simulink model "Quat"  (R2022b)
settings: Solver=FixedStepAuto  StartTime=0.0  StopTime=10.0  RelTol=1e-3
settings Model: Creator=yuzehong  LastModifiedBy=程一帆
settings OptimizationCC: DefaultParameterBehavior=Inlined  UseDivisionForNetSlopeComputation=on  GainParamInheritBuiltInType=on  UseFloatMulNetSlope=on  InlineInvariantSignals=on  ReuseModelBlockBuffer=on  PassReuseOutputArgsAs=Individual arguments  NoFixptDivByZeroProtection=on  EfficientFloat2IntCast=on  LifeSpan=1  OptimizeBlockOrder=speed  DifferentSizesBufferReuse=on  EfficientTunableParamExpr=on
settings DebuggingCC: ParameterTunabilityLossMsg=error
settings HardwareCC: ProdLongLongMode=on
settings SFSimCC: MATLABDynamicMemAlloc=off
settings RTWCC: Description=Embedded Coder  SystemTargetFile=ert.tlc  GenCodeOnly=on  TemplateMakefile=ert_default_tmf  GPUComputeCapability=5.0
settings CodeAppCC: GenerateComments=off  IgnoreCustomStorageClasses=off  OperatorAnnotations=on  SimulinkDataObjDesc=on  SFDataObjDesc=on  CustomSymbolStrGlobalVar=rt$N$M  CustomSymbolStrType=$N$M  CustomSymbolStrFcn=$N$M$F  CustomSymbolStrMacro=$N$M  SimulinkBlockComments=off
settings ERTTargetCC: TargetLangStandard=C99 (ISO)  GenerateSampleERTMain=on  IncludeMdlTerminateFcn=off  CombineSignalStateStructs=on  SupportAbsoluteTime=off  CodeInterfacePackaging=Reusable function  SupportComplex=off  SupportContinuousTime=on  InlinedParameterPlacement=NonHierarchical  ERTCustomFileTemplate=example_file_process.tlc  ERTFilePackagingFormat=CompactWithDataFile

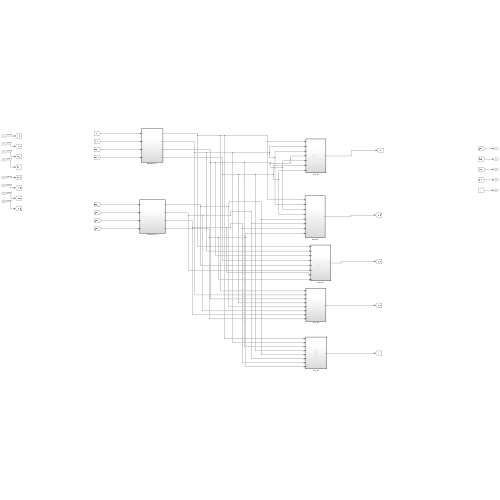
[thumbnail: Simulink's stored preview of the top-level diagram]
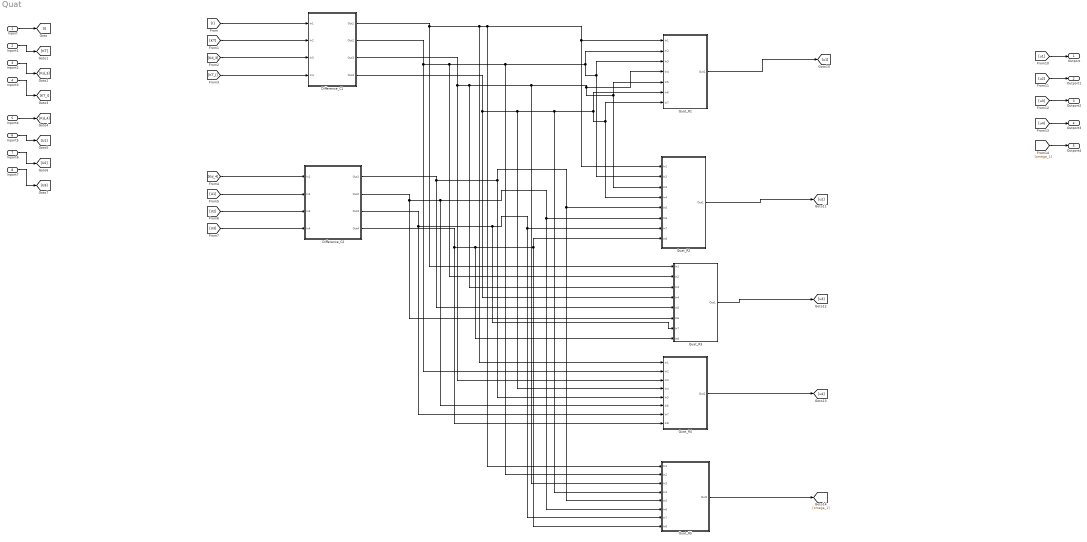
== system Quat ==
  Inport : Inport  OutDataTypeStr=int32  PortDimensions=8
  Inport1 : Inport  Port=2  OutDataTypeStr=int32  PortDimensions=8
  Inport2 : Inport  Port=3  OutDataTypeStr=int32  PortDimensions=8
  Inport3 : Inport  Port=4  OutDataTypeStr=int32  PortDimensions=8
  Inport4 : Inport  Port=5  OutDataTypeStr=int32  PortDimensions=8
  Inport5 : Inport  Port=6  OutDataTypeStr=int32  PortDimensions=8
  Inport6 : Inport  Port=7  OutDataTypeStr=int32  PortDimensions=8
  Inport7 : Inport  Port=8  OutDataTypeStr=int32  PortDimensions=8
  Difference_C1 : Subsystem  TreatAsAtomicUnit=on
      settings: RTWFcnNameOpts=Use subsystem name
  Difference_C2 : Subsystem  TreatAsAtomicUnit=on
      settings: RTWFcnNameOpts=Use subsystem name
  Quat_R1 : Subsystem  TreatAsAtomicUnit=on
      settings: RTWFcnNameOpts=Use subsystem name
  Quat_R2 : Subsystem  TreatAsAtomicUnit=on
      settings: RTWFcnNameOpts=Use subsystem name
  Quat_R3 : Subsystem  TreatAsAtomicUnit=on
      settings: RTWFcnNameOpts=Use subsystem name
  Quat_R4 : Subsystem  TreatAsAtomicUnit=on
      settings: RTWFcnNameOpts=Use subsystem name
  Quat_R5 : Subsystem  TreatAsAtomicUnit=on
      settings: RTWFcnNameOpts=Use subsystem name
  Outport : Outport
  Outport1 : Outport  Port=2
  Outport2 : Outport  Port=3
  Outport3 : Outport  Port=4
  Outport4 : Outport  Port=5
  wires:
  Quat_R1/1(Out1) -> [u1]
  Quat_R2/1(Out1) -> [u2]
  Quat_R3/1(Out1) -> [u3]
  Quat_R4/1(Out1) -> [u4]
  Quat_R5/1(Out1) -> [omega_1]
  Difference_C1/3(Out3) -> Quat_R4/3(In3), Quat_R3/3(In3), Quat_R5/3(In3), Quat_R1/4(In4), Quat_R2/3(In3), Quat_R1/5(In5)
  Difference_C1/2(Out2) -> Quat_R4/2(In2), Quat_R3/2(In2), Quat_R5/2(In2), Quat_R1/2(In2), Quat_R2/2(In2), Quat_R1/3(In3)
  Difference_C1/4(Out4) -> Quat_R3/4(In4), Quat_R4/4(In4), Quat_R5/4(In4), Quat_R1/6(In6), Quat_R2/4(In4), Quat_R1/7(In7)
  Difference_C1/1(Out1) -> Quat_R3/1(In1), Quat_R4/1(In1), Quat_R5/1(In1), Quat_R2/1(In1), Quat_R1/1(In1)
  [I] -> Difference_C1/1(In1)
  [KT] -> Difference_C1/2(In2)
  [Kd_3] -> Difference_C1/3(In3)
  [KT_I] -> Difference_C1/4(In4)
  Difference_C2/4(Out4) -> Quat_R4/8(In8), Quat_R3/8(In8), Quat_R5/8(In8), Quat_R2/8(In8)
  Difference_C2/2(Out2) -> Quat_R3/6(In6), Quat_R4/6(In6), Quat_R5/6(In6), Quat_R2/6(In6)
  Difference_C2/3(Out3) -> Quat_R4/7(In7), Quat_R3/7(In7), Quat_R5/7(In7), Quat_R2/7(In7)
  Difference_C2/1(Out1) -> Quat_R3/5(In5), Quat_R4/5(In5), Quat_R5/5(In5), Quat_R2/5(In5)
  [Kd_4] -> Difference_C2/1(In1)
  [U1] -> Difference_C2/2(In2)
  [U2] -> Difference_C2/3(In3)
  [U3] -> Difference_C2/4(In4)
  Inport/1 -> [I]
  Inport1/1 -> [KT]
  Inport2/1 -> [Kd_3]
  Inport3/1 -> [KT_I]
  Inport4/1 -> [Kd_4]
  Inport5/1 -> [U1]
  Inport6/1 -> [U2]
  Inport7/1 -> [U3]
  [u1] -> Outport/1
  [u2] -> Outport1/1
  [u3] -> Outport2/1
  [u4] -> Outport3/1
  [omega_1] -> Outport4/1

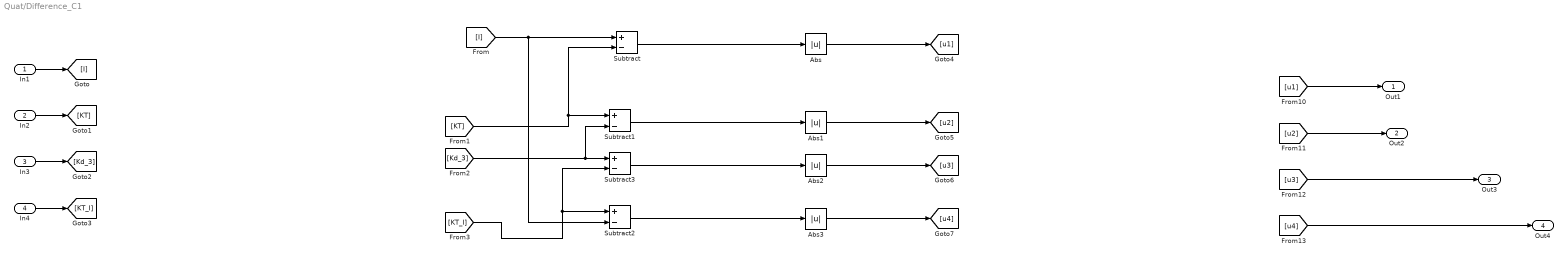
== system Quat/Difference_C1 ==
  In1 : Inport
  In2 : Inport  Port=2
  In3 : Inport  Port=3
  In4 : Inport  Port=4
  Abs{,1..3} (4 alike) : Abs  SaturateOnIntegerOverflow=off
  Subtract{,1..3} (4 alike) : Sum  Inputs=+-
  Out1 : Outport
  Out2 : Outport  Port=2
  Out3 : Outport  Port=3
  Out4 : Outport  Port=4
  wires:
  [KT_I] -> Subtract3/2, Subtract2/1
  Subtract2/1 -> Abs3/1
  [I] -> Subtract2/2, Subtract/1
  [Kd_3] -> Subtract1/2, Subtract3/1
  Subtract1/1 -> Abs1/1
  [KT] -> Subtract/2, Subtract1/1
  Subtract/1 -> Abs/1
  Abs1/1 -> [u2]
  Subtract3/1 -> Abs2/1
  Abs/1 -> [u1]
  In1/1 -> [I]
  In2/1 -> [KT]
  In3/1 -> [Kd_3]
  In4/1 -> [KT_I]
  [u3] -> Out3/1
  [u4] -> Out4/1
  [u1] -> Out1/1
  [u2] -> Out2/1
  Abs2/1 -> [u3]
  Abs3/1 -> [u4]

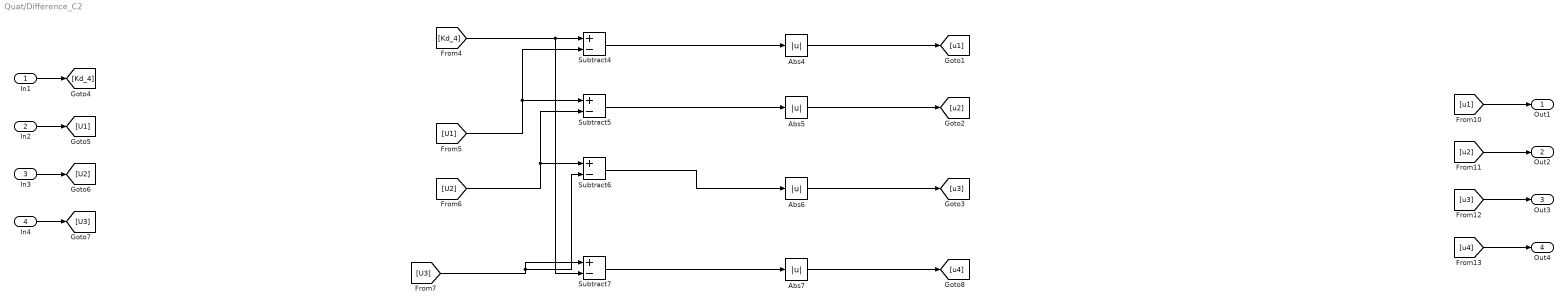
== system Quat/Difference_C2 ==
  In1 : Inport
  In2 : Inport  Port=2
  In3 : Inport  Port=3
  In4 : Inport  Port=4
  Abs{4..7} (4 alike) : Abs  SaturateOnIntegerOverflow=off
  Subtract{4..7} (4 alike) : Sum  Inputs=+-
  Out1 : Outport
  Out2 : Outport  Port=2
  Out3 : Outport  Port=3
  Out4 : Outport  Port=4
  wires:
  Subtract5/1 -> Abs5/1
  [U3] -> Subtract7/1, Subtract6/2
  Subtract6/1 -> Abs6/1
  [U2] -> Subtract5/2, Subtract6/1
  [Kd_4] -> Subtract7/2, Subtract4/1
  [U1] -> Subtract4/2, Subtract5/1
  Subtract7/1 -> Abs7/1
  Subtract4/1 -> Abs4/1
  Abs5/1 -> [u2]
  Abs6/1 -> [u3]
  Abs4/1 -> [u1]
  Abs7/1 -> [u4]
  In1/1 -> [Kd_4]
  In2/1 -> [U1]
  In3/1 -> [U2]
  In4/1 -> [U3]
  [u1] -> Out1/1
  [u2] -> Out2/1
  [u3] -> Out3/1
  [u4] -> Out4/1

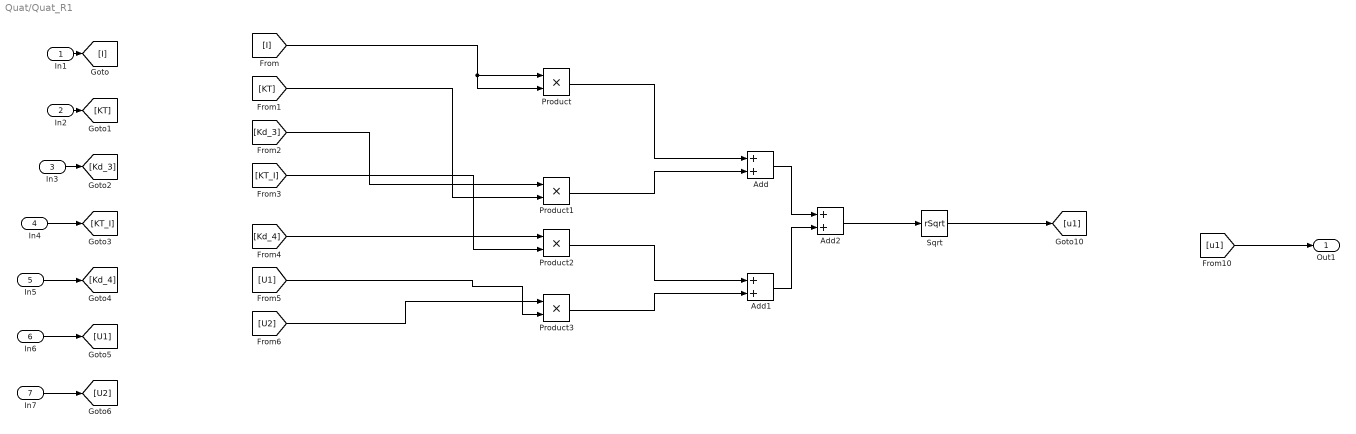
== system Quat/Quat_R1 ==
  In1 : Inport
  In2 : Inport  Port=2
  In3 : Inport  Port=3
  In4 : Inport  Port=4
  In5 : Inport  Port=5
  In6 : Inport  Port=6
  In7 : Inport  Port=7
  Add : Sum  SaturateOnIntegerOverflow=on
  Add1 : Sum  SaturateOnIntegerOverflow=on
  Add2 : Sum  SaturateOnIntegerOverflow=on
  Product{,1..3} (4 alike) : Product  OutDataTypeStr=int32
  Sqrt : Sqrt  Operator=rSqrt  OutDataTypeStr=single  SaturateOnIntegerOverflow=off
  Out1 : Outport
  wires:
  Product3/1 -> Add1/2
  Product1/1 -> Add/2
  Product/1 -> Add/1
  Add/1 -> Add2/1
  [I] -> Product/2, Product/1
  Add1/1 -> Add2/2
  Product2/1 -> Add1/1
  Add2/1 -> Sqrt/1
  Sqrt/1 -> [u1]
  [KT] -> Product1/2
  [Kd_3] -> Product1/1
  [U2] -> Product3/1
  [U1] -> Product3/2
  [KT_I] -> Product2/2
  [Kd_4] -> Product2/1
  In1/1 -> [I]
  In2/1 -> [KT]
  In3/1 -> [Kd_3]
  In4/1 -> [KT_I]
  In5/1 -> [Kd_4]
  In6/1 -> [U1]
  In7/1 -> [U2]
  [u1] -> Out1/1

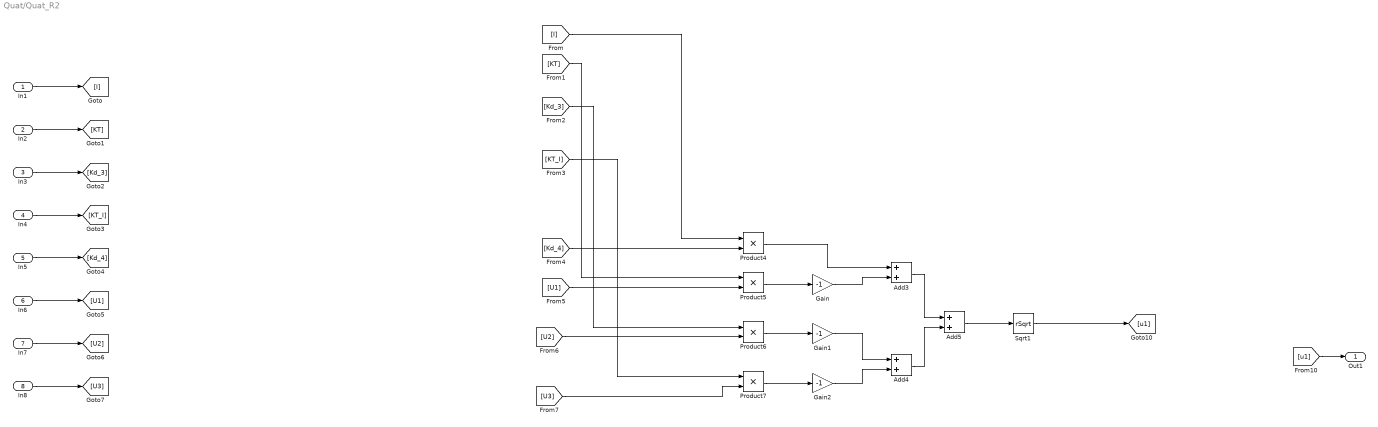
== system Quat/Quat_R2 ==
  In1 : Inport
  In2 : Inport  Port=2
  In3 : Inport  Port=3
  In4 : Inport  Port=4
  In5 : Inport  Port=5
  In6 : Inport  Port=6
  In7 : Inport  Port=7
  In8 : Inport  Port=8
  Add3 : Sum  OutDataTypeStr=int32  SaturateOnIntegerOverflow=on
  Add4 : Sum  SaturateOnIntegerOverflow=on
  Add5 : Sum  SaturateOnIntegerOverflow=on
  Gain : Gain  Gain=-1  OutDataTypeStr=int32
  Gain1 : Gain  Gain=-1  OutDataTypeStr=int32
  Gain2 : Gain  Gain=-1  OutDataTypeStr=int32
  Product{4..7} (4 alike) : Product  OutDataTypeStr=int32
  Sqrt1 : Sqrt  Operator=rSqrt  OutDataTypeStr=single  SaturateOnIntegerOverflow=off
  Out1 : Outport
  wires:
  Product7/1 -> Gain2/1
  Gain/1 -> Add3/2
  Add4/1 -> Add5/2
  Product4/1 -> Add3/1
  Gain2/1 -> Add4/2
  Gain1/1 -> Add4/1
  Product6/1 -> Gain1/1
  Product5/1 -> Gain/1
  Add5/1 -> Sqrt1/1
  Add3/1 -> Add5/1
  [KT_I] -> Product7/1
  Sqrt1/1 -> [u1]
  [U1] -> Product5/2
  [Kd_3] -> Product6/1
  [U2] -> Product6/2
  [Kd_4] -> Product4/2
  [U3] -> Product7/2
  [I] -> Product4/1
  [KT] -> Product5/1
  In1/1 -> [I]
  In2/1 -> [KT]
  In3/1 -> [Kd_3]
  In4/1 -> [KT_I]
  In5/1 -> [Kd_4]
  In6/1 -> [U1]
  In7/1 -> [U2]
  In8/1 -> [U3]
  [u1] -> Out1/1

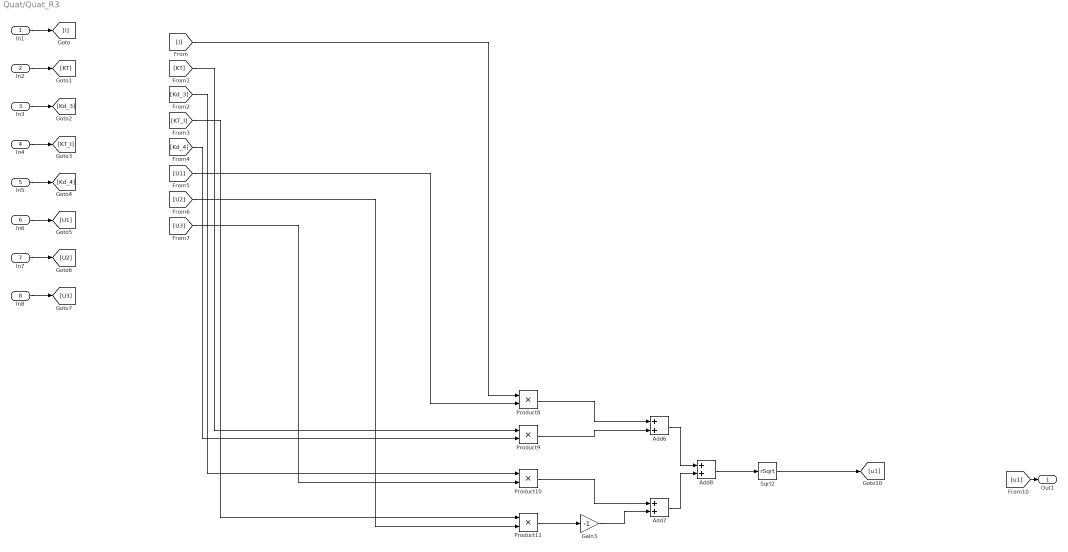
== system Quat/Quat_R3 ==
  In1 : Inport
  In2 : Inport  Port=2
  In3 : Inport  Port=3
  In4 : Inport  Port=4
  In5 : Inport  Port=5
  In6 : Inport  Port=6
  In7 : Inport  Port=7
  In8 : Inport  Port=8
  Add6 : Sum  OutDataTypeStr=int32  SaturateOnIntegerOverflow=on
  Add7 : Sum  OutDataTypeStr=int32  SaturateOnIntegerOverflow=on
  Add8 : Sum  OutDataTypeStr=int32  SaturateOnIntegerOverflow=on
  Gain3 : Gain  Gain=-1  OutDataTypeStr=int32
  Product{8..11} (4 alike) : Product  OutDataTypeStr=int32
  Sqrt2 : Sqrt  Operator=rSqrt  OutDataTypeStr=single  SaturateOnIntegerOverflow=off
  Out1 : Outport
  wires:
  Product8/1 -> Add6/1
  [U3] -> Product10/2
  Add7/1 -> Add8/2
  Add8/1 -> Sqrt2/1
  [I] -> Product8/1
  Product9/1 -> Add6/2
  [U1] -> Product8/2
  Product10/1 -> Add7/1
  Product11/1 -> Gain3/1
  Gain3/1 -> Add7/2
  [KT] -> Product9/1
  Add6/1 -> Add8/1
  [Kd_3] -> Product10/1
  [KT_I] -> Product11/1
  [U2] -> Product11/2
  Sqrt2/1 -> [u1]
  [Kd_4] -> Product9/2
  In1/1 -> [I]
  In2/1 -> [KT]
  In3/1 -> [Kd_3]
  In4/1 -> [KT_I]
  In5/1 -> [Kd_4]
  In6/1 -> [U1]
  In7/1 -> [U2]
  In8/1 -> [U3]
  [u1] -> Out1/1

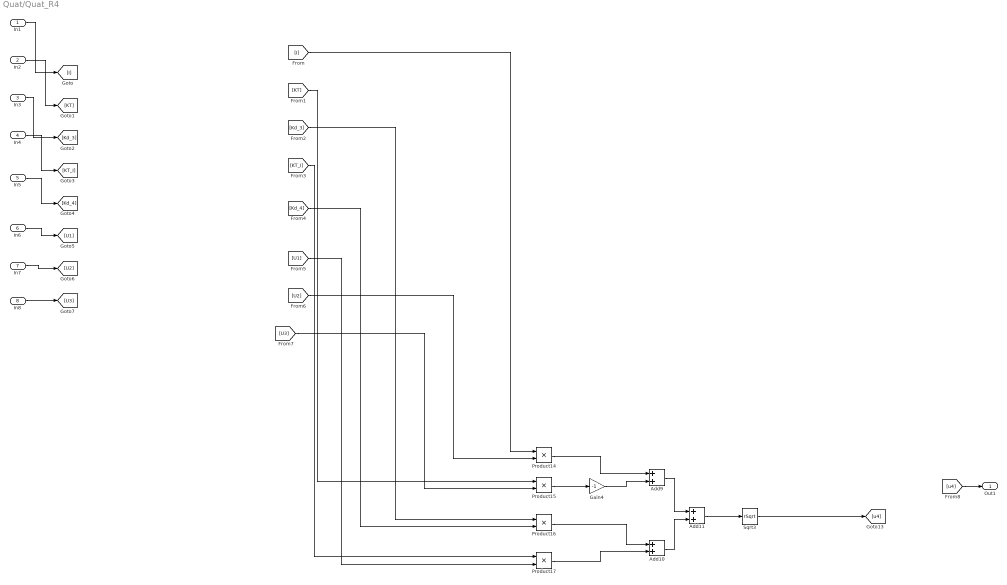
== system Quat/Quat_R4 ==
  In1 : Inport
  In2 : Inport  Port=2
  In3 : Inport  Port=3
  In4 : Inport  Port=4
  In5 : Inport  Port=5
  In6 : Inport  Port=6
  In7 : Inport  Port=7
  In8 : Inport  Port=8
  Add10 : Sum  SaturateOnIntegerOverflow=on
  Add11 : Sum  SaturateOnIntegerOverflow=on
  Add9 : Sum  OutDataTypeStr=int32  SaturateOnIntegerOverflow=on
  Gain4 : Gain  Gain=-1  OutDataTypeStr=int32
  Product{14..17} (4 alike) : Product  OutDataTypeStr=int32
  Sqrt3 : Sqrt  Operator=rSqrt  OutDataTypeStr=single  SaturateOnIntegerOverflow=off
  Out1 : Outport
  wires:
  [U2] -> Product14/2
  Add11/1 -> Sqrt3/1
  Add10/1 -> Add11/2
  Product15/1 -> Gain4/1
  [Kd_3] -> Product16/1
  Product17/1 -> Add10/2
  [Kd_4] -> Product16/2
  Gain4/1 -> Add9/2
  Product16/1 -> Add10/1
  Add9/1 -> Add11/1
  Product14/1 -> Add9/1
  [U1] -> Product17/2
  [KT] -> Product15/1
  Sqrt3/1 -> [u4]
  [KT_I] -> Product17/1
  [I] -> Product14/1
  [U3] -> Product15/2
  In1/1 -> [I]
  In2/1 -> [KT]
  In3/1 -> [Kd_3]
  In4/1 -> [KT_I]
  In5/1 -> [Kd_4]
  In6/1 -> [U1]
  In7/1 -> [U2]
  In8/1 -> [U3]
  [u4] -> Out1/1

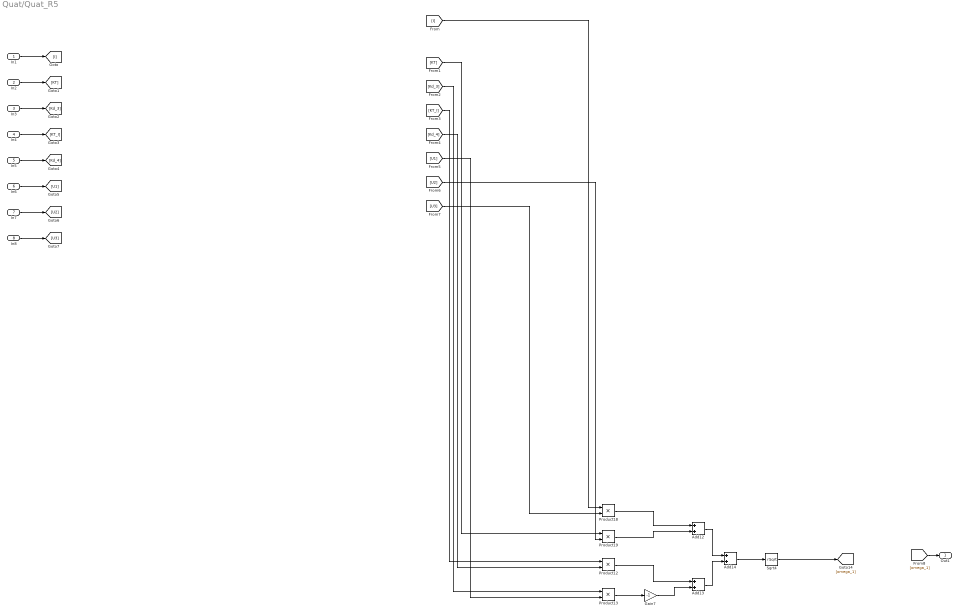
== system Quat/Quat_R5 ==
  In1 : Inport
  In2 : Inport  Port=2
  In3 : Inport  Port=3
  In4 : Inport  Port=4
  In5 : Inport  Port=5
  In6 : Inport  Port=6
  In7 : Inport  Port=7
  In8 : Inport  Port=8
  Add12 : Sum  SaturateOnIntegerOverflow=on
  Add13 : Sum  OutDataTypeStr=int32  SaturateOnIntegerOverflow=on
  Add14 : Sum  OutDataTypeStr=int32  SaturateOnIntegerOverflow=on
  Gain7 : Gain  Gain=-1  OutDataTypeStr=int32
  Product{12..13,18..19} (4 alike) : Product  OutDataTypeStr=int32
  Sqrt4 : Sqrt  Operator=rSqrt  OutDataTypeStr=single  SaturateOnIntegerOverflow=off
  Out1 : Outport
  wires:
  Product18/1 -> Add12/1
  Product19/1 -> Add12/2
  Add12/1 -> Add14/1
  Product12/1 -> Add13/1
  [KT_I] -> Product12/1
  Gain7/1 -> Add13/2
  Product13/1 -> Gain7/1
  Add13/1 -> Add14/2
  Add14/1 -> Sqrt4/1
  [KT] -> Product19/1
  [Kd_3] -> Product13/1
  [Kd_4] -> Product12/2
  [I] -> Product18/1
  [U3] -> Product18/2
  Sqrt4/1 -> [omega_1]
  [U2] -> Product19/2
  [U1] -> Product13/2
  In1/1 -> [I]
  In2/1 -> [KT]
  In3/1 -> [Kd_3]
  In4/1 -> [KT_I]
  In5/1 -> [Kd_4]
  In6/1 -> [U1]
  In7/1 -> [U2]
  In8/1 -> [U3]
  [omega_1] -> Out1/1
